simulink model "SIR_Italy_VariableBetaGamma100_R2019b"  (R2019b)
settings: Solver=FixedStepAuto  StartTime=0.0  StopTime=180  FixedStep=0.001  RelTol=1e-9  AbsTol=1e-9
undefined symbols (not defined in the file): a, beta1, beta2, beta3, g, gamma1, gamma2, gamma3, I0, P, R0, st3
libraries: fuzblock x3
settings Model: OrderedModelArguments=off  Creator=ismae  LastModifiedBy=ismae
settings SolverCC: SolverResetMethod=Robust

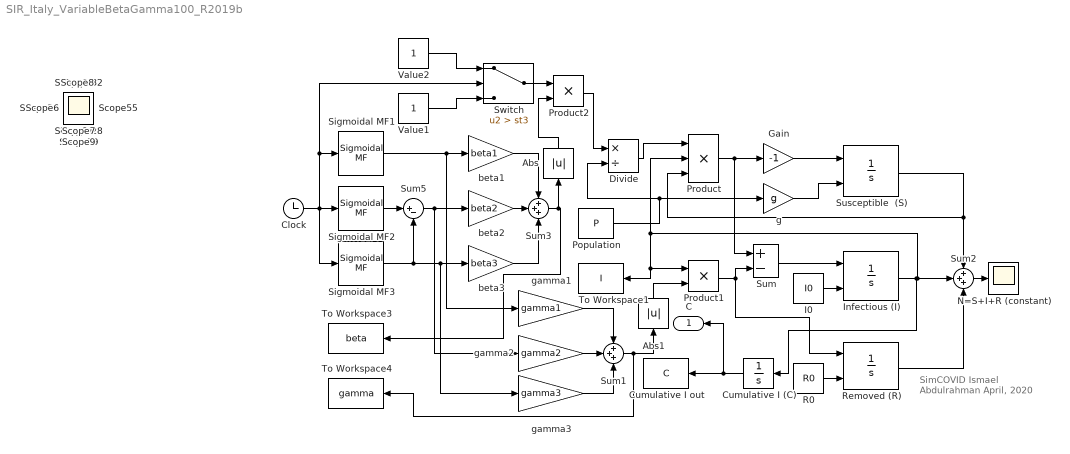
== system SIR_Italy_VariableBetaGamma100_R2019b ==
  note: SimCOVID
      | Ismael Abdulrahman
      | April, 2020
  Abs : Abs
  Abs1 : Abs
  Clock : Clock
  Cumulative I (C) : Integrator
  Cumulative I out : ToWorkspace  VariableName=C  SampleTime=-1
      settings: Save2DSignal=2-D array (concatenate along first dimension)
  Divide : Product  Inputs=*/
  Gain : Gain  Gain=-1
  I0 : Constant  Value=I0
  Infectious (I) : Integrator  InitialConditionSource=external
  N=S+I+R (constant) : Scope
  Population : Constant  Value=P
  Product : Product  Inputs=3
  Product1 : Product
  Product2 : Product
  R0 : Constant  Value=R0
  Removed (R) : Integrator  InitialConditionSource=external
  Sigmoidal MF1 : fuzblock/Membership  Functions/Sigmoidal MF  a=-a  c=st1
      settings: SourceProductBaseCode=FL
  Sigmoidal MF2 : fuzblock/Membership  Functions/Sigmoidal MF  a=a  c=st1
      settings: SourceProductBaseCode=FL
  Sigmoidal MF3 : fuzblock/Membership  Functions/Sigmoidal MF  a=a  c=st2
      settings: SourceProductBaseCode=FL
  Sum : Sum  Inputs=+-
  Sum1 : Sum  Inputs=+++
  Sum2 : Sum  Inputs=+++
  Sum3 : Sum  Inputs=+++
  Sum5 : Sum  Inputs=|+-
  Susceptible  (S) : Integrator  InitialConditionSource=external  InitialCondition=10000
  Switch : Switch  Criteria=u2 > Threshold  Threshold=st3
  To Workspace1 : ToWorkspace  VariableName=I  SampleTime=-1
      settings: Save2DSignal=2-D array (concatenate along first dimension)
  To Workspace3 : ToWorkspace  VariableName=beta  SampleTime=-1
      settings: Save2DSignal=2-D array (concatenate along first dimension)
  To Workspace4 : ToWorkspace  VariableName=gamma  SampleTime=-1
      settings: Save2DSignal=2-D array (concatenate along first dimension)
  Value1 : Constant
  Value2 : Constant
  beta1 : Gain  Gain=beta1
  beta2 : Gain  Gain=beta2
  beta3 : Gain  Gain=beta3
  g : Gain  Gain=g
  gamma1 : Gain  Gain=gamma1
  gamma2 : Gain  Gain=gamma2
  gamma3 : Gain  Gain=gamma3
  C : Outport
  Scope{,1..32} (33 alike) : Scope
  wires:
  Product/1 -> Gain/1, Sum/1
  Divide/1 -> Product/1
  Sum/1 -> Infectious (I)/1
  I0/1 -> Infectious (I)/2
  Population/1 -> Divide/2, g/1
  Sum2/1 -> N=S+I+R (constant)/1
  R0/1 -> Removed (R)/2
  Product1/1 -> Removed (R)/1, Sum/2
  beta3/1 -> Sum3/3
  beta2/1 -> Sum3/2
  beta1/1 -> Sum3/1
  Susceptible  (S)/1 -> Product/3, Sum2/1
  Gain/1 -> Susceptible  (S)/1
  Removed (R)/1 -> Sum2/3
  Cumulative I (C)/1 -> Cumulative I out/1, C/1
  Sum1/1 -> Abs1/1, To Workspace4/1
  Sigmoidal MF1/1 -> gamma1/1, beta1/1
  Sigmoidal MF2/1 -> Sum5/1
  gamma1/1 -> Sum1/1
  Sigmoidal MF3/1 -> gamma3/1, beta3/1, Sum5/2
  Sum5/1 -> gamma2/1, beta2/1
  gamma3/1 -> Sum1/3
  gamma2/1 -> Sum1/2
  Infectious (I)/1 -> Product1/1, To Workspace1/1, Product/2, Sum2/2, Cumulative I (C)/1
  g/1 -> Susceptible  (S)/2
  Sum3/1 -> To Workspace3/1, Abs/1
  Value1/1 -> Switch/3
  Switch/1 -> Product2/1
  Value2/1 -> Switch/1
  Clock/1 -> Sigmoidal MF1/1, Switch/2, Sigmoidal MF2/1, Sigmoidal MF3/1
  Product2/1 -> Divide/1
  Abs/1 -> Product2/2
  Abs1/1 -> Product1/2
